simulink model "DiagnosticsLogger"  (R2024a)
settings: Solver=VariableStepAuto  StartTime=0.0  StopTime=10.0  RelTol=1e-3
settings Model: DataDictionary=BMS_System_Arch_dict.sldd  Creator=ghourabi  LastModifiedBy=ghourabi

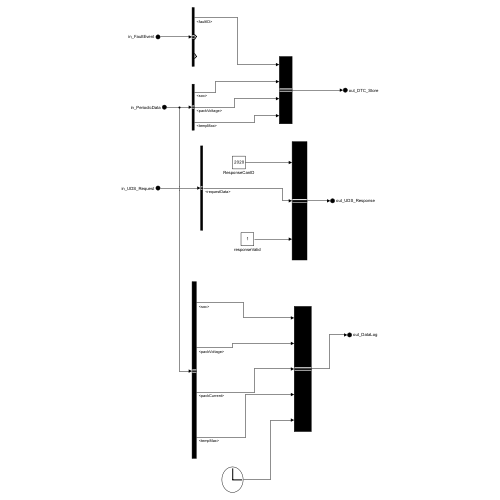
[thumbnail: Simulink's stored preview of the top-level diagram]
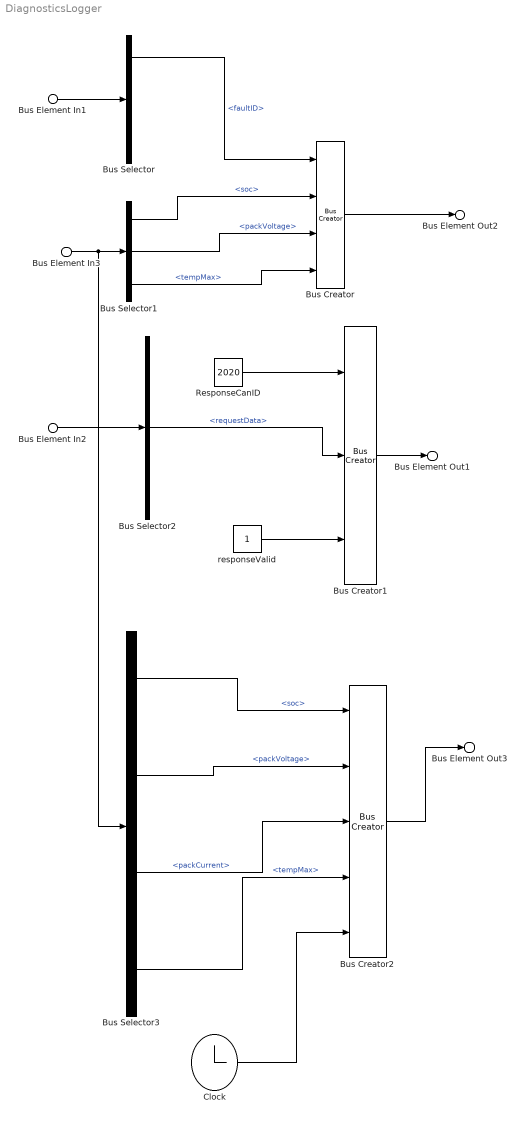
== system DiagnosticsLogger ==
  Bus Element In1 : Inport  PortName=in_FaultEvent
  Bus Element In2 : Inport  Port=2  PortName=in_UDS_Request
  Bus Element In3 : Inport  Port=3  PortName=in_PeriodicData
  Bus Creator : BusCreator  Inputs=4
  Bus Creator1 : BusCreator  Inputs=3
  Bus Creator2 : BusCreator  Inputs=5
  Bus Selector : BusSelector  OutputSignals=faultID,faultSeverity,faultTimestamp
  Bus Selector1 : BusSelector  OutputSignals=soc,packVoltage,tempMax
  Bus Selector2 : BusSelector  OutputSignals=requestData
  Bus Selector3 : BusSelector  OutputSignals=soc,packVoltage,packCurrent,tempMax
  Clock : Clock
      settings: Decimation=1000
  ResponseCanID : Constant  Value=2020
  responseValid : Constant
  Bus Element Out1 : Outport  PortName=out_UDS_Response
  Bus Element Out2 : Outport  Port=2  PortName=out_DTC_Store
  Bus Element Out3 : Outport  Port=3  PortName=out_DataLog
  wires:
  Bus Element In1/1 -> Bus Selector/1
  Bus Element In3/1 -> Bus Selector3/1, Bus Selector1/1
  Bus Selector/1 -> Bus Creator/1  "<faultID>"
  Bus Selector1/1 -> Bus Creator/2  "<soc>"
  Bus Selector1/2 -> Bus Creator/3  "<packVoltage>"
  Bus Selector1/3 -> Bus Creator/4  "<tempMax>"
  Bus Creator/1 -> Bus Element Out2/1
  Bus Element In2/1 -> Bus Selector2/1
  Bus Selector2/1 -> Bus Creator1/2  "<requestData>"
  Bus Creator1/1 -> Bus Element Out1/1
  ResponseCanID/1 -> Bus Creator1/1
  responseValid/1 -> Bus Creator1/3
  Bus Selector3/1 -> Bus Creator2/1  "<soc>"
  Bus Selector3/2 -> Bus Creator2/2  "<packVoltage>"
  Bus Selector3/3 -> Bus Creator2/3  "<packCurrent>"
  Bus Selector3/4 -> Bus Creator2/4  "<tempMax>"
  Clock/1 -> Bus Creator2/5
  Bus Creator2/1 -> Bus Element Out3/1
